simulink model "kyvadloMPCaKF"  (R2018a)
settings: Solver=VariableStepAuto  StartTime=0.0  StopTime=10  MaxStep=0.01  RelTol=1e-3  EnableMultiTasking=on
PreLoadFcn:
  | m1=0.4;        % Hmotnost vozika [kg]
  | m2=0.08;      % Hmotnost kyvadla [kg]
  | l=0.2;            % Vzdialenost taziska od osi rotacie [m]
  | g=9.81;         % Tiazove zrychlenie [m/s2]
  | b=0.1;           % Koeficient trenia [m/s]
StartFcn:
  | kyvadloOfflineMPCaKF
values from neighbouring files (symbols this model uses):
  A = bus.a    [.m]    (also in MPCjedenkrok.m; MPCuzavretaslucka.m; inkrementalny.m; kombinovaneobmedzenia.m)
  Ac = -1/tau    (= -0.0166666666667)    [integrator.m]    (also in obmedzenia.m = [Acu;Acx]; stavovyprikaz.m = [-0.313 56.7 0; -0.0139 -0.426 0; 0 56.7 0]; testrozsirenieintegrator.m)
  B = bus.b(:,2)    [.m]    (also in MPCjedenkrok.m; MPCuzavretaslucka.m; inkrementalny.m; kombinovaneobmedzenia.m)
  b0 = [b0u; b0x]    [obmedzenia.m]
  B0 = [zeros(2*p5*nu,nx); B0x]    [obmedzenia.m]
  C = bus.c    [.m]    (also in MPCjedenkrok.m; MPCuzavretaslucka.m; inkrementalny.m; kombinovaneobmedzenia.m)
  G = G+N((i-1)*nx+1:i*nx,:)'*P*M((i-1)*nx+1:i*nx,:)    [ucelovafunkcia.m]
  H = (H+H')/2    [.m]    (also in MPCuzavretaslucka.m; inkrementalny.m; integrator.m; kombinovaneobmedzenia.m)
  Rf = diag(v_var)    [kyvadloOfflineMPCaKF.m]
  Ts = 5    [integrator.m]    (also in kyvadloOfflineLQ.m = kyvadlo.Ts; kyvadloOfflineMPC.m = kyvadlo.Ts; kyvadloOfflineMPCaKF.m = kyvadlo.Ts; stavovyprikaz.m = 0.5)
  uh = 0.002    [.m]    (also in MPCjedenkrok.m = 0.01; MPCuzavretaslucka.m = 0.01; integrator.m = 10; kombinovaneobmedzenia.m = 0.005)
  ul = -uh    (= -0.01)    [MPCjedenkrok.m]    (also in MPCuzavretaslucka.m; integrator.m = 0; kyvadloOfflineLQ.m = -5; kyvadloOfflineMPC.m = -5)
  v_var = [1e-3 1e-3]'    [kyvadloOfflineMPCaKF.m]
  w_var = [0 0 0 1e-5]'    [kyvadloOfflineMPCaKF.m]
  x1h = 0.5    [kyvadloOfflineLQ.m]    (also in kyvadloOfflineMPC.m; kyvadloOfflineMPCaKF.m)
  x1l = -x1h    (= -0.5)    [kyvadloOfflineLQ.m]    (also in kyvadloOfflineMPC.m; kyvadloOfflineMPCaKF.m)
undefined symbols (not defined in the file or in its folder): Discrete, Time
libraries: simulink x2, ctrlSharedLib x1
settings Model: Creator=UAMAI-LENOVO  LastModifiedBy=Gergely
settings DataIOCC: LimitDataPoints=on  SaveFormat=Array
settings OptimizationCC: LifeSpan=inf
settings DebuggingCC: SFUnexpectedBacktrackingDiag=warning  SFNoUnconditionalDefaultTransitionDiag=warning  SFExecutionAtInitializationDiag=none
settings HardwareCC: ProdBitPerPointer=32  ProdBitPerSizeT=32  ProdBitPerPtrDiffT=32  ProdLargestAtomicFloat=None  ProdIntDivRoundTo=Undefined  ProdEndianess=Unspecified  ProdWordSize=32  ProdHWDeviceType=32-bit Generic
settings ModelReferenceCC: PropagateSignalLabelsOutOfModel=off
settings CodeAppCC: StateflowObjectComments=on
settings GRTTargetCC: TargetLangStandard=C89/C90 (ANSI)  GeneratePreprocessorConditionals=Disable all
settings ConfigComp: CovMetricSettings=dw  CovHtmlReporting=on  CovSaveCumulativeToWorkspaceVar=on  CovSaveSingleToWorkspaceVar=on  CovExternalEMLEnable=off

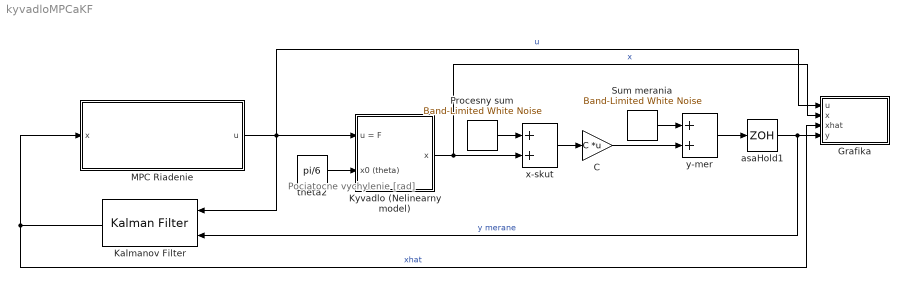
== system kyvadloMPCaKF ==
  note: Pociatocne
      | vychylenie [rad]
  " y-mer " : Sum
  C : Gain  Gain=C  Multiplication=Matrix(K*u)
  Grafika : Subsystem
  Kalmanov Filter : ctrlSharedLib/Kalman Filter  TimeDomain=Discrete-Time  UseCurrentEstimator=on  ModelSource=Individual A, B, C, D matrices  ModelSourceVariable=kyvadlo  A=A  B=B  C=C  D=0  NumberOfStates=1  NumberOfInputs=1  NumberOfOutputs=1  InitialEstimateSource=Dialog  X0=0  P0=10  UseK=off  UseGH=off  NumberOfProcessNoiseInputs=1  G=1  TimeInvariantG=on  H=0  TimeInvariantH=on  Q=Qf  TimeInvariantQ=on  R=Rf  TimeInvariantR=on  N=0  TimeInvariantN=on  AddInputPort=on  AddEnablePort=off  OutputEstimatedY=off  OutputP=off  Ts=Ts
      settings: SourceProductBaseCode=CT
  Kyvadlo (Nelinearny model) : Subsystem
  MPC Riadenie : Subsystem
  Procesny sum : simulink/Sources/Band-Limited White Noise  Cov=w_var*Ts  Ts=Ts  seed=[23341]
  Sum merania : simulink/Sources/Band-Limited White Noise  Cov=v_var*Ts  Ts=Ts  seed=[12347]
  asaHold1 : ZeroOrderHold  SampleTime=Ts
  theta2 : Constant  Value=pi/6
  x-skut : Sum
  wires:
  theta2/1 -> Kyvadlo (Nelinearny model)/2(x0 (theta))
  Kyvadlo (Nelinearny model)/1(x) -> x-skut/2, Grafika/2(x)  "x"
  Sum merania/1 -> " y-mer "/1
  C/1 -> " y-mer "/2
  Procesny sum/1 -> x-skut/1
  x-skut/1 -> C/1
  " y-mer "/1 -> asaHold1/1
  Kalmanov Filter/1 -> Grafika/3(xhat), MPC Riadenie/1(x)  "xhat"
  asaHold1/1 -> Grafika/4(y), Kalmanov Filter/2  "y merane"
  MPC Riadenie/1(u) -> Kyvadlo (Nelinearny model)/1(u = F), Grafika/1(u), Kalmanov Filter/1  "u"

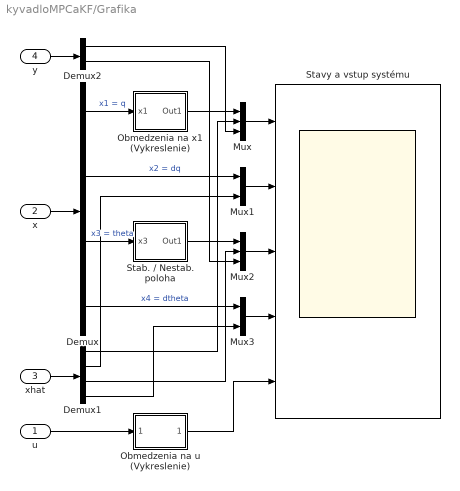
== system kyvadloMPCaKF/Grafika ==
  u : Inport
  x : Inport  Port=2
  xhat : Inport  Port=3
  y : Inport  Port=4
  " Stavy a vstup systému" : Scope  NumInputPorts=5
  Demux : Demux
  Demux1 : Demux
  Demux2 : Demux  Outputs=2
  Mux : Mux  Inputs=3
  Mux1 : Mux  Inputs=2
  Mux2 : Mux  Inputs=3
  Mux3 : Mux  Inputs=2
  Obmedzenia na u (Vykreslenie) : Subsystem
  "Obmedzenia na x1 (Vykreslenie) " : Subsystem
  Stab. / Nestab. poloha : Subsystem
  wires:
  Demux/3 -> Stab. / Nestab. poloha/1(x3)  "x3 = theta"
  u/1 -> Obmedzenia na u (Vykreslenie)/1(u = F)
  Demux/1 -> "Obmedzenia na x1 (Vykreslenie) "/1(x1)  "x1 = q"
  x/1 -> Demux/1
  Obmedzenia na u (Vykreslenie)/1(Out1) -> " Stavy a vstup systému"/5
  xhat/1 -> Demux1/1
  Mux/1 -> " Stavy a vstup systému"/1
  "Obmedzenia na x1 (Vykreslenie) "/1(Out1) -> Mux/1
  Demux1/1 -> Mux/2
  Demux/2 -> Mux1/1  "x2 = dq"
  Demux1/2 -> Mux1/2
  Mux1/1 -> " Stavy a vstup systému"/2
  Stab. / Nestab. poloha/1(Out1) -> Mux2/1
  Demux1/3 -> Mux2/2
  Mux2/1 -> " Stavy a vstup systému"/3
  Demux/4 -> Mux3/1  "x4 = dtheta"
  Mux3/1 -> " Stavy a vstup systému"/4
  Demux1/4 -> Mux3/2
  y/1 -> Demux2/1
  Demux2/1 -> Mux/3
  Demux2/2 -> Mux2/3

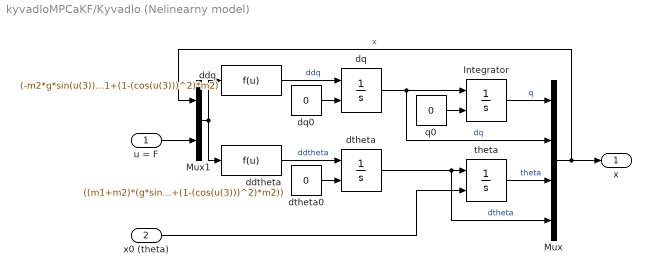
== system kyvadloMPCaKF/Kyvadlo (Nelinearny model) ==
  u = F : Inport
  x0 (theta) : Inport  Port=2
  Integrator : Integrator  InitialConditionSource=external
  Mux : Mux
  Mux1 : Mux  Inputs=2
  ddq : Fcn  Expr=(-m2*g*sin(u(3))*cos(u(3))+m2*l*((u(4))^2)*sin(u(3))+b*m2*u(4)*cos(u(3))+u(5))/(m1+(1-(cos(u(3)))^2)*m2)
  ddtheta : Fcn  Expr=((m1+m2)*(g*sin(u(3))-b*u(4))-(m2*l*((u(4))^2)*sin(u(3))+u(5))*cos(u(3)))/(l*(m1+(1-(cos(u(3)))^2)*m2))
  dq : Integrator  InitialConditionSource=external
  dq0 : Constant  Value=0
  dtheta : Integrator  InitialConditionSource=external
  dtheta0 : Constant  Value=0
  q0 : Constant  Value=0
  theta : Integrator  InitialConditionSource=external
  x : Outport
  wires:
  Mux/1 -> x/1, Mux1/1  "x"
  ddq/1 -> dq/1  "ddq"
  dq/1 -> Mux/2, Integrator/1  "dq"
  ddtheta/1 -> dtheta/1  "ddtheta"
  x0 (theta)/1 -> theta/2
  q0/1 -> Integrator/2
  Integrator/1 -> Mux/1  "q"
  theta/1 -> Mux/3  "theta"
  dtheta/1 -> Mux/4, theta/1  "dtheta"
  Mux1/1 -> ddtheta/1, ddq/1
  dq0/1 -> dq/2
  dtheta0/1 -> dtheta/2
  u = F/1 -> Mux1/2

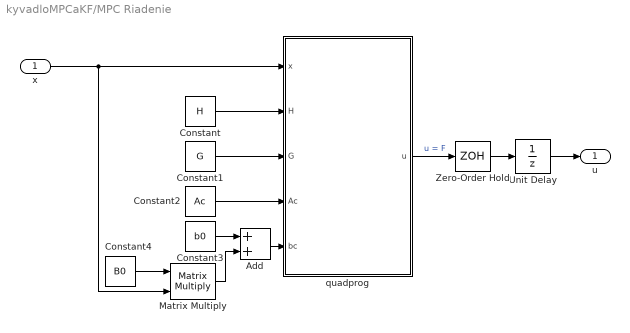
== system kyvadloMPCaKF/MPC Riadenie ==
  x : Inport
  Add : Sum
  Constant : Constant  Value=H
  Constant1 : Constant  Value=G
  Constant2 : Constant  Value=Ac
  Constant3 : Constant  Value=b0
  Constant4 : Constant  Value=B0
  Matrix Multiply : Product  Multiplication=Matrix(*)
  Unit Delay : UnitDelay  SampleTime=-1
  Zero-Order Hold : ZeroOrderHold  SampleTime=Ts
  quadprog : MATLAB Function  TreatAsAtomicUnit=on
  u : Outport
  wires:
  Matrix Multiply/1 -> Add/2
  Add/1 -> quadprog/5(bc)
  Constant3/1 -> Add/1
  Constant2/1 -> quadprog/4(Ac)
  Constant/1 -> quadprog/2(H)
  x/1 -> Matrix Multiply/2, quadprog/1(x)
  Constant1/1 -> quadprog/3(G)
  quadprog/1(u) -> Zero-Order Hold/1  "u = F"
  Constant4/1 -> Matrix Multiply/1
  Zero-Order Hold/1 -> Unit Delay/1
  Unit Delay/1 -> u/1

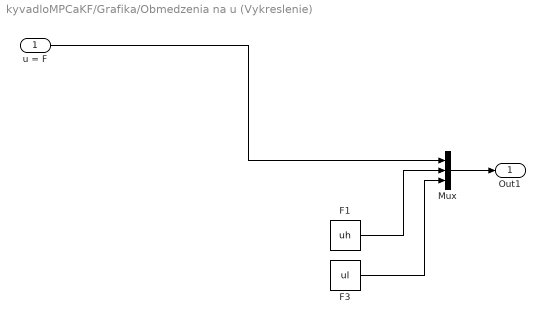
== system kyvadloMPCaKF/Grafika/Obmedzenia na u (Vykreslenie) ==
  u = F : Inport
  F1 : Constant  Value=uh
  F3 : Constant  Value=ul
  Mux : Mux  Inputs=3
  Out1 : Outport
  wires:
  F1/1 -> Mux/2
  F3/1 -> Mux/3
  u = F/1 -> Mux/1
  Mux/1 -> Out1/1

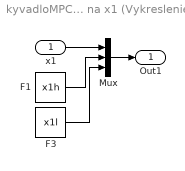
== system kyvadloMPCaKF/Grafika/Obmedzenia na x1 (Vykreslenie)  ==
  x1 : Inport
  F1 : Constant  Value=x1h
  F3 : Constant  Value=x1l
  Mux : Mux  Inputs=3
  Out1 : Outport
  wires:
  F1/1 -> Mux/2
  F3/1 -> Mux/3
  x1/1 -> Mux/1
  Mux/1 -> Out1/1

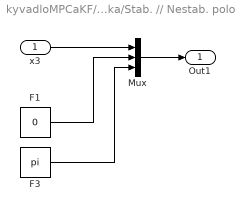
== system kyvadloMPCaKF/Grafika/Stab. // Nestab. poloha ==
  x3 : Inport
  F1 : Constant  Value=0
  F3 : Constant  Value=pi
  Mux : Mux  Inputs=3
  Out1 : Outport
  wires:
  F1/1 -> Mux/2
  F3/1 -> Mux/3
  x3/1 -> Mux/1
  Mux/1 -> Out1/1

== matlab function kyvadloMPCaKF/MPC Riadenie/quadprog ==
  data: x input; u output; H input; G input; Ac input; bc input
function u  = qp(x,H,G,Ac,bc)      % Riesenie QP  
    u=0;                           % Inicializacia
    coder.extrinsic('optimoptions')% Neexistuje C verzia
    coder.extrinsic('quadprog');   % Neexistuje C verzia
    o=optimoptions('quadprog','Display','none');% Vypnut 
    U=quadprog(H,G*x,Ac,bc,[],[],[],[],[],o); % Volanie
    u = U(1);                      % Vystup
